simulink model "PID_Controller"  (R2020b)
settings: Solver=VariableStepAuto  StartTime=0.0  StopTime=0.1  RelTol=1e-3
values from neighbouring files (symbols this model uses):
  Kd = 0.15    [initial_values.sldd]
  Ki = 500.0    [initial_values.sldd]
  Kp = 21.0    [initial_values.sldd]
settings Model: DataDictionary=initial_values.sldd  Creator=Vrunda M Balgi  LastModifiedBy=Vrunda M Balgi
settings DataIOCC: SaveOutput=off  SaveTime=off

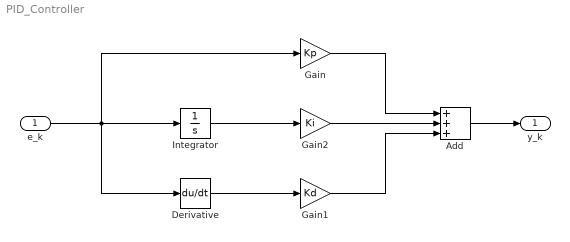
== system PID_Controller ==
  e_k : Inport  OutDataTypeStr=double  PortDimensions=1  SampleTime=0
  Add : Sum  Inputs=+++
  Derivative : Derivative
  Gain : Gain  Gain=Kp
  Gain1 : Gain  Gain=Kd
  Gain2 : Gain  Gain=Ki
  Integrator : Integrator
  y_k : Outport  OutDataTypeStr=double  PortDimensions=1  SampleTime=0
  wires:
  e_k/1 -> Integrator/1, Gain/1, Derivative/1
  Gain/1 -> Add/1
  Gain2/1 -> Add/2
  Gain1/1 -> Add/3
  Derivative/1 -> Gain1/1
  Integrator/1 -> Gain2/1
  Add/1 -> y_k/1
